simulink model "Full_scale_sim"  (R2024b)
settings: Solver=VariableStepAuto  StartTime=0.0  StopTime=60  RelTol=1e-3
values from neighbouring files (symbols this model uses):
  A_adrcl = [zeros(N, 1)  eye(N, N) ... (first row only)    [Control_Full_Scale_init_example_single_blade_installation.m]
  A_o = [A_m e_m*c_T_d_m ... (first row only)    [Control_Full_Scale_init_example_single_blade_installation.m]
  A_o_lqr = [A_m_lqr e_m*c_T_d_m_lqr ... (first row only)    [Control_Full_Scale_init_example_single_blade_installation.m]
  A_o_nmlqr = [A_m_nmlqr e_m*c_T_d_m_nmlqr ... (first row only)    [Control_Full_Scale_init_example_single_blade_installation.m]
  A_o_plqr = A_m_lqr    [Control_Full_Scale_init_example_single_blade_installation.m]
  b0 = 9.345442381739944e-04    (= 0.000934544238174)    [Control_Full_Scale_init_example_single_blade_installation.m]
  b_adrcl = [zeros(N-1, 1) ... (first row only)    [Control_Full_Scale_init_example_single_blade_installation.m]
  b_o = [b_m ... (first row only)    [Control_Full_Scale_init_example_single_blade_installation.m]
  b_o_lqr = [b_m_lqr ... (first row only)    [Control_Full_Scale_init_example_single_blade_installation.m]
  b_o_nmlqr = [b_m_nmlqr ... (first row only)    [Control_Full_Scale_init_example_single_blade_installation.m]
  b_o_plqr = b_m_lqr    [Control_Full_Scale_init_example_single_blade_installation.m]
  c_o_T = [c_T_m 0]    [Control_Full_Scale_init_example_single_blade_installation.m]
  c_o_T_lqr = [c_T_m_lqr 0]    [Control_Full_Scale_init_example_single_blade_installation.m]
  c_o_T_nmlqr = [c_T_m_nmlqr 0]    [Control_Full_Scale_init_example_single_blade_installation.m]
  c_o_T_plqr = c_T_m_lqr    [Control_Full_Scale_init_example_single_blade_installation.m]
  c_t = [1, zeros(1, N)]    [Control_Full_Scale_init_example_single_blade_installation.m]
  damping_en = 1    [Control_Full_Scale_init_example_single_blade_installation.m]
  eta_init_n = [p_init_n;Theta_init_n]    [Control_Full_Scale_init_example_single_blade_installation.m]
  k = ones(N,1)    [Control_Full_Scale_init_example_single_blade_installation.m]
  k_c_T = acker(A_m,b_m, [-omega_cl,-omega_cl])    [Control_Full_Scale_init_example_single_blade_installation.m]
  k_c_T_lqr = lqr(A_m_lqr,b_m_lqr,Q,R)    [Control_Full_Scale_init_example_single_blade_installation.m]
  k_c_T_nmlqr = lqr(A_m_nmlqr,b_m_nmlqr,Q,R)    [Control_Full_Scale_init_example_single_blade_installation.m]
  k_d_T = (e_m*c_T_d_m) \ b_m    [Control_Full_Scale_init_example_single_blade_installation.m]
  k_d_T_lqr = (e_m*c_T_d_m_lqr) \ b_m_lqr    [Control_Full_Scale_init_example_single_blade_installation.m]
  k_d_T_nmlqr = (e_m*c_T_d_m_nmlqr) \ b_m_nmlqr    [Control_Full_Scale_init_example_single_blade_installation.m]
  k_o = acker(A_o',c_o_T',[-omega_O,-omega_O,-omega_O])'    [Control_Full_Scale_init_example_single_blade_installation.m]
  k_o_lqr = acker(A_o_lqr',c_o_T_lqr',[-omega_O,-omega_O,-omega_O])'    [Control_Full_Scale_init_example_single_blade_installation.m]
  k_o_nmlqr = acker(A_o_nmlqr',c_o_T_nmlqr',[-omega_O,-omega_O,-omega_O])'    [Control_Full_Scale_init_example_single_blade_installation.m]
  k_o_plqr = acker(A_o_plqr',c_o_T_plqr',[-omega_O,-omega_O])'    [Control_Full_Scale_init_example_single_blade_installation.m]
  k_plqr = lqr(A_m_lqr, b_m_lqr, Q, R)    [Control_Full_Scale_init_example_single_blade_installation.m]
  k_s = -inv(c_T_m*inv(A_m-b_m*k_c_T)*b_m)    [Control_Full_Scale_init_example_single_blade_installation.m]
  k_s_lqr = -inv(c_T_m_lqr*inv(A_m_lqr-b_m_lqr*k_c_T_lqr)*b_m_lqr)    [Control_Full_Scale_init_example_single_blade_installation.m]
  k_s_nmlqr = -inv(c_T_m_nmlqr*inv(A_m_nmlqr-b_m_nmlqr*k_c_T_nmlqr)*b_m_nmlqr)    [Control_Full_Scale_init_example_single_blade_installation.m]
  k_s_plqr = -inv(c_T_m*inv(A_m-b_m*k_plqr)*b_m)    [Control_Full_Scale_init_example_single_blade_installation.m]
  k_w1 = gamma * EA/lw1_init    (= 68722339.2973)    [Control_Full_Scale_init_example_single_blade_installation.m]
  k_w2 = 1e8    (= 100000000)    [Control_Full_Scale_init_example_single_blade_installation.m]
  l = ones(N+1, 1)    [Control_Full_Scale_init_example_single_blade_installation.m]
  LADRC_max_effort = 900    [Control_Full_Scale_init_example_single_blade_installation.m]
  lw2 = norm(p_h_init- posSling_n(:,1))-elong_lw2    [Control_Full_Scale_init_example_single_blade_installation.m]
  meanWindSpeed = 12    [Control_Full_Scale_init_example_single_blade_installation.m]
  N = 2    [Control_Full_Scale_init_example_single_blade_installation.m]
  nu_init_b = zeros(6,1)    [Control_Full_Scale_init_example_single_blade_installation.m]
  pitch_damping = 100e+3    (= 100000)    [Control_Full_Scale_init_example_single_blade_installation.m]
  posCraneTip = [0;0;-110]    [Control_Full_Scale_init_example_single_blade_installation.m]
  posSling_b = [bladePar.posCOG + [slings_p1_new(1); -4.5; slings_p1_new(2)],                 bladePar.posCOG + [slings_p1_new(1); 4.5; slings_p1_new(2)],                bladePar.posCOG + [slings_p2_new(1); -4.5; slings_p2_new(2)],                bladePar.posCOG + [slings_p2_new(1); 4.5; slings_p2_new(2)]]    [Control_Full_Scale_init_example_single_blade_installation.m]
  posTuggerline_b = [bladePar.posCOG+[0;-4.5;0],bladePar.posCOG+[0;-35;0]]    [Control_Full_Scale_init_example_single_blade_installation.m]
undefined symbols (not defined in the file or in its folder): bladePar, k_T_d, sigbuilder_block
libraries: MarIn_blade x24, simulink_extras x3, vrlib x3, slpidlib x2, dspstat3 x1
(part 1 of 2)
settings Model: Creator=Basti  LastModifiedBy=Henrik
settings DebuggingCC: UnconnectedInputMsg=warning  UnconnectedOutputMsg=warning  UnconnectedLineMsg=warning
settings ModelReferenceCC: EnableRefExpFcnMdlSchedulingChecks=on
settings RTWCC: GPUComputeCapability=3.5  DLArmComputeVersion=19.05

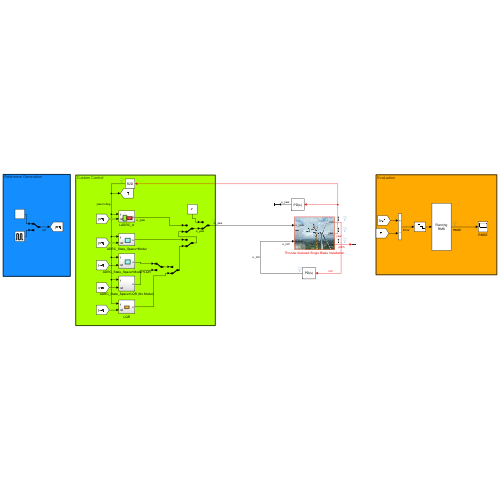
[thumbnail: Simulink's stored preview of the top-level diagram]
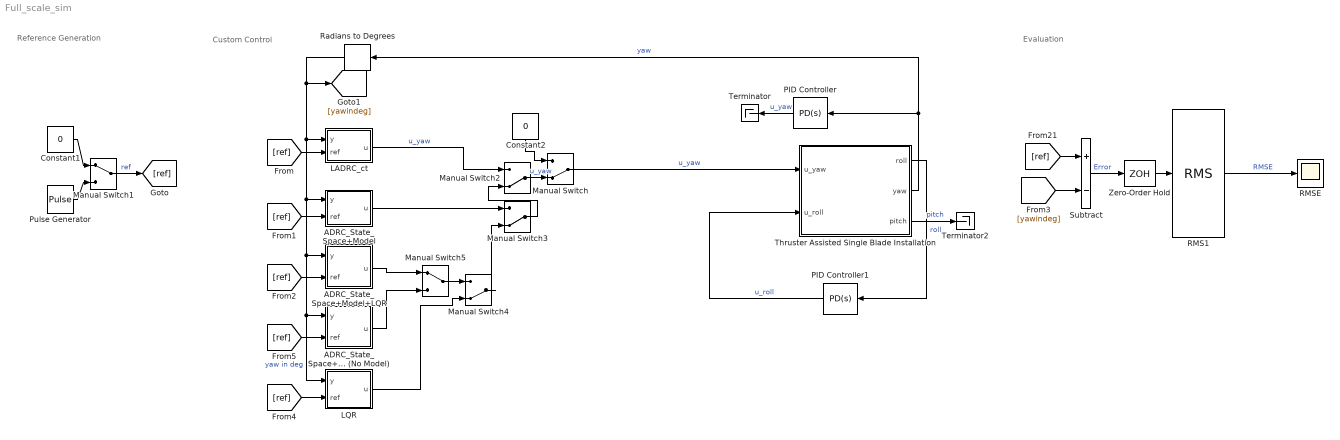
== system Full_scale_sim ==
  note: Evaluation
  note: Reference Generation
  note: Custom Control
  ADRC_State_Space+LQR (No Model) : Subsystem
  ADRC_State_Space+Model : Subsystem
  ADRC_State_Space+Model+LQR : Subsystem
  Constant1 : Constant  Value=0
  Constant2 : Constant  Value=0
  LADRC_ct : Subsystem
  LQR : Subsystem
  Manual Switch{,2..4} (4 alike) : ManualSwitch  CurrentSetting=0
  Manual Switch1 : ManualSwitch
  Manual Switch5 : ManualSwitch
  PID Controller : slpidlib/PID Controller  Controller=PD  Form=Parallel  TimeDomain=Continuous-time  UseExternalTs=off  SampleTime=-1  IntegratorMethod=Forward Euler  FilterMethod=Forward Euler  ControllerParametersSource=internal  P=5000  I=0  UseKiTs=off  D=35414.6651049002  UseExternalDerivativeSource=off  N=35.5205953021552  UseFilter=on  TunerSelectOption=Transfer Function Based (PID Tuner App)  InitialConditionSource=internal  InitialConditionForIntegrator=0  InitialConditionForFilter=0  DifferentiatorICPrevScaledInput=0  ExternalReset=none  TrackingMode=off  Kt=1  LimitOutput=off  SatLimitsSource=internal  UpperSaturationLimit=inf  LowerSaturationLimit=-inf  LinearizeAsGain=on  AntiWindupMode=none  Kb=1  LimitIntegrator=off  UpperIntegratorSaturationLimit=inf  LowerIntegratorSaturationLimit=-inf  POutMin=[]  POutMax=[]  IOutMin=[]  IOutMax=[]  DOutMin=[]  DOutMax=[]  NOutMin=[]  NOutMax=[]  SumOutMin=[]  SumOutMax=[]  SaturationOutMin=[]  SaturationOutMax=[]  PParamMin=[]  PParamMax=[]  IParamMin=[]  IParamMax=[]  DParamMin=[]  DParamMax=[]  NParamMin=[]  NParamMax=[]  KbParamMin=[]  KbParamMax=[]  KtParamMin=[]  KtParamMax=[]  KbOutMin=[]  KbOutMax=[]  KtOutMin=[]  KtOutMax=[]  IntegratorOutMin=[]  IntegratorOutMax=[]  FilterOutMin=[]  FilterOutMax=[]  SumI1OutMin=[]  SumI1OutMax=[]  SumI2OutMin=[]  SumI2OutMax=[]  SumI3OutMin=[]  SumI3OutMax=[]  SumI4OutMin=[]  SumI4OutMax=[]  SumDOutMin=[]  SumDOutMax=[]  DifferentiatorOutMin=[]  DifferentiatorOutMax=[]  FilterDiffOutCoefMin=[]  FilterDiffOutCoefMax=[]  ReciprocalOutMin=[]  ReciprocalOutMax=[]  SumDenOutMin=[]  SumDenOutMax=[]  SumNumOutMin=[]  SumNumOutMax=[]  DivideOutMin=[]  DivideOutMax=[]  UdiffTsProdOutMin=[]  UdiffTsProdOutMax=[]  NTsProdOutMin=[]  NTsProdOutMax=[]  UintegralTsProdOutMin=[]  UintegralTsProdOutMax=[]  UngainTsProdOutMin=[]  UngainTsProdOutMax=[]  ClampingZeroOutDataTypeStr=Inherit: Inherit via back propagation  ClampingZeroOutMin=[]  ClampingZeroOutMax=[]  FilterDenConstantOutDataTypeStr=Inherit: Inherit via back propagation  FilterDenConstantOutMin=[]  FilterDenConstantOutMax=[]  PCopyOutDataTypeStr=Inherit: Inherit via back propagation  PCopyOutMin=[]  PCopyOutMax=[]  NCopyOutDataTypeStr=Inherit: Inherit via back propagation  NCopyOutMin=[]  NCopyOutMax=[]  IntegratorContinuousStateAttributes=''  IntegratorStateMustResolveToSignalObject=off  IntegratorRTWStateStorageClass=Auto  FilterContinuousStateAttributes=''  FilterStateMustResolveToSignalObject=off  FilterRTWStateStorageClass=Auto  ParallelPVariant=InternalParameters  IdealPVariant=Disabled  IVariant=Disabled  DVariant=InternalParameters  IntegratorVariant=Disabled  SatVariant=Disabled  AWVariant=Disabled  PCopyVariant=Disabled  TRVariant=Disabled  FdbkBlocksVariant=Forward  IdealPFdbkVariant=Disabled  SatFdbkVariant=Disabled  DerivativeFilterVariant=ContFilter  NVariant=InternalParameters  NCopyVariant=Disabled  FilterICVariant=InternalICsFilter  IntegratorICVariant=Disabled  ExternalResetVariant=Disabled  TRSumVariant=Passthrough  SumFdbkVariant=Disabled  SumVariant=Sum_PD  TsampFilterVariant=InternalTs  TsampNgainVariant=Passthrough  TsampIntegralVariant=Disabled_SignalSpec  ExternalSaturationOutDataTypeStr=Inherit: Same as second input  DerivativeSourceVariant=ErrorSignal  PreIntVariant=InternalPreInt
  PID Controller1 : slpidlib/PID Controller  Controller=PD  Form=Parallel  TimeDomain=Continuous-time  UseExternalTs=off  SampleTime=-1  IntegratorMethod=Forward Euler  FilterMethod=Forward Euler  ControllerParametersSource=internal  P=200  I=0  UseKiTs=off  D=300000  UseExternalDerivativeSource=off  N=100  UseFilter=on  TunerSelectOption=Transfer Function Based (PID Tuner App)  InitialConditionSource=internal  InitialConditionForIntegrator=0  InitialConditionForFilter=0  DifferentiatorICPrevScaledInput=0  ExternalReset=none  TrackingMode=off  Kt=1  LimitOutput=off  SatLimitsSource=internal  UpperSaturationLimit=inf  LowerSaturationLimit=-inf  LinearizeAsGain=on  AntiWindupMode=none  Kb=1  LimitIntegrator=off  UpperIntegratorSaturationLimit=inf  LowerIntegratorSaturationLimit=-inf  POutMin=[]  POutMax=[]  IOutMin=[]  IOutMax=[]  DOutMin=[]  DOutMax=[]  NOutMin=[]  NOutMax=[]  SumOutMin=[]  SumOutMax=[]  SaturationOutMin=[]  SaturationOutMax=[]  PParamMin=[]  PParamMax=[]  IParamMin=[]  IParamMax=[]  DParamMin=[]  DParamMax=[]  NParamMin=[]  NParamMax=[]  KbParamMin=[]  KbParamMax=[]  KtParamMin=[]  KtParamMax=[]  KbOutMin=[]  KbOutMax=[]  KtOutMin=[]  KtOutMax=[]  IntegratorOutMin=[]  IntegratorOutMax=[]  FilterOutMin=[]  FilterOutMax=[]  SumI1OutMin=[]  SumI1OutMax=[]  SumI2OutMin=[]  SumI2OutMax=[]  SumI3OutMin=[]  SumI3OutMax=[]  SumI4OutMin=[]  SumI4OutMax=[]  SumDOutMin=[]  SumDOutMax=[]  DifferentiatorOutMin=[]  DifferentiatorOutMax=[]  FilterDiffOutCoefMin=[]  FilterDiffOutCoefMax=[]  ReciprocalOutMin=[]  ReciprocalOutMax=[]  SumDenOutMin=[]  SumDenOutMax=[]  SumNumOutMin=[]  SumNumOutMax=[]  DivideOutMin=[]  DivideOutMax=[]  UdiffTsProdOutMin=[]  UdiffTsProdOutMax=[]  NTsProdOutMin=[]  NTsProdOutMax=[]  UintegralTsProdOutMin=[]  UintegralTsProdOutMax=[]  UngainTsProdOutMin=[]  UngainTsProdOutMax=[]  ClampingZeroOutDataTypeStr=Inherit: Inherit via back propagation  ClampingZeroOutMin=[]  ClampingZeroOutMax=[]  FilterDenConstantOutDataTypeStr=Inherit: Inherit via back propagation  FilterDenConstantOutMin=[]  FilterDenConstantOutMax=[]  PCopyOutDataTypeStr=Inherit: Inherit via back propagation  PCopyOutMin=[]  PCopyOutMax=[]  NCopyOutDataTypeStr=Inherit: Inherit via back propagation  NCopyOutMin=[]  NCopyOutMax=[]  IntegratorContinuousStateAttributes=''  IntegratorStateMustResolveToSignalObject=off  IntegratorRTWStateStorageClass=Auto  FilterContinuousStateAttributes=''  FilterStateMustResolveToSignalObject=off  FilterRTWStateStorageClass=Auto  ParallelPVariant=InternalParameters  IdealPVariant=Disabled  IVariant=Disabled  DVariant=InternalParameters  IntegratorVariant=Disabled  SatVariant=Disabled  AWVariant=Disabled  PCopyVariant=Disabled  TRVariant=Disabled  FdbkBlocksVariant=Forward  IdealPFdbkVariant=Disabled  SatFdbkVariant=Disabled  DerivativeFilterVariant=ContFilter  NVariant=InternalParameters  NCopyVariant=Disabled  FilterICVariant=InternalICsFilter  IntegratorICVariant=Disabled  ExternalResetVariant=Disabled  TRSumVariant=Passthrough  SumFdbkVariant=Disabled  SumVariant=Sum_PD  TsampFilterVariant=InternalTs  TsampNgainVariant=Passthrough  TsampIntegralVariant=Disabled_SignalSpec  ExternalSaturationOutDataTypeStr=Inherit: Same as second input  DerivativeSourceVariant=ErrorSignal  PreIntVariant=InternalPreInt
  Pulse Generator : DiscretePulseGenerator  PulseType=Time based  Amplitude=90  Period=40  PulseWidth=50
  RMS1 : dspstat3/RMS  run=on  directionMode=Entire input  dimension=1  reset_popup=None
  RMSE : Scope
  Radians to Degrees : simulink_extras/Transformations/Radians to Degrees
  Subtract : Sum  Inputs=+-
  Terminator : Terminator
  Terminator2 : Terminator
  Thruster Assisted Single Blade Installation : Subsystem  AncestorBlock=MarIn_blade/[Example] Single blade installation  mask([Example] Single blade installation){}
      mask help:
      | This is an example to use the MarIn toolbox to model single blade installation.
      |
      | Author: Zhengru Ren
      | Date:  19/09/2017
      mask Display: image('apsicon.png');
  Zero-Order Hold : ZeroOrderHold  SampleTime=0.5
  wires:
  Thruster Assisted Single Blade Installation/3(pitch) -> Terminator2/1  "pitch"
  Thruster Assisted Single Blade Installation/2(yaw) -> Radians to Degrees/1, PID Controller/1  "yaw"
  PID Controller1/1 -> Thruster Assisted Single Blade Installation/2(u_roll)  "u_roll"
  Thruster Assisted Single Blade Installation/1(roll) -> PID Controller1/1  "roll"
  Manual Switch/1 -> Thruster Assisted Single Blade Installation/1(u_yaw)  "u_yaw"
  PID Controller/1 -> Terminator/1  "u_yaw"
  Radians to Degrees/1 -> LQR/1(y), ADRC_State_Space+LQR (No Model)/1(y), ADRC_State_Space+Model+LQR/1(y), ADRC_State_Space+Model/1(y), LADRC_ct/1(y), [yawindeg]  "yaw in deg"
  LADRC_ct/1(u) -> Manual Switch2/1  "u_yaw"
  ADRC_State_Space+Model/1(u) -> Manual Switch3/1
  Constant1/1 -> Manual Switch1/1
  Pulse Generator/1 -> Manual Switch1/2
  Manual Switch2/1 -> Manual Switch/2  "u_yaw"
  Constant2/1 -> Manual Switch/1
  Subtract/1 -> Zero-Order Hold/1  "Error"
  [ref] -> Subtract/1
  RMS1/1 -> RMSE/1  "RMSE"
  Manual Switch1/1 -> [ref]  "ref"
  [ref] -> LADRC_ct/2(ref)
  [ref] -> ADRC_State_Space+Model/2(ref)
  [ref] -> ADRC_State_Space+Model+LQR/2(ref)
  ADRC_State_Space+Model+LQR/1(u) -> Manual Switch5/1
  Manual Switch3/1 -> Manual Switch2/2
  Zero-Order Hold/1 -> RMS1/1
  [yawindeg] -> Subtract/2
  [ref] -> LQR/2(ref)
  LQR/1(u) -> Manual Switch4/2
  Manual Switch4/1 -> Manual Switch3/2
  [ref] -> ADRC_State_Space+LQR (No Model)/2(ref)
  ADRC_State_Space+LQR (No Model)/1(u) -> Manual Switch5/2
  Manual Switch5/1 -> Manual Switch4/1

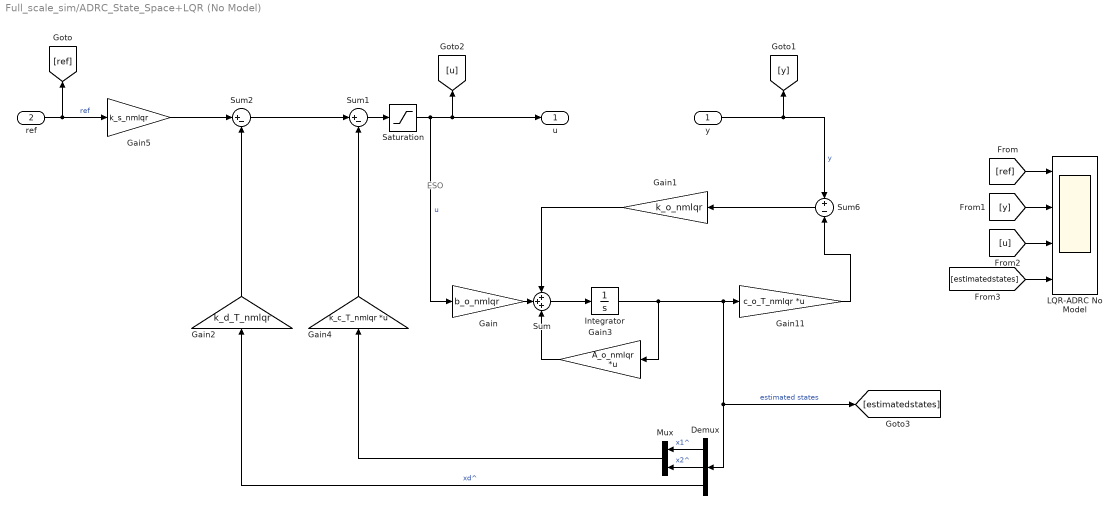
== system Full_scale_sim/ADRC_State_Space+LQR (No Model) ==
  note: ESO
  y : Inport
  ref : Inport  Port=2
  Demux : Demux  Outputs=N+1
  Gain : Gain  Gain=b_o_nmlqr
  Gain1 : Gain  Gain=k_o_nmlqr
  Gain11 : Gain  Gain=c_o_T_nmlqr  Multiplication=Matrix(K*u)
  Gain2 : Gain  Gain=k_d_T_nmlqr
  Gain3 : Gain  Gain=A_o_nmlqr  Multiplication=Matrix(K*u)
  Gain4 : Gain  Gain=k_c_T_nmlqr  Multiplication=Matrix(K*u)
  Gain5 : Gain  Gain=k_s_nmlqr
  Integrator : Integrator
  LQR-ADRC No Model : Scope  NumInputPorts=4
  Mux : Mux  Inputs=2
  Saturation : Saturate  UpperLimit=LADRC_max_effort  LowerLimit=-LADRC_max_effort
  Sum : Sum  Inputs=+++
  Sum1 : Sum  Inputs=|+-
  Sum2 : Sum  Inputs=|+-
  Sum6 : Sum  Inputs=+|-
  u : Outport
  wires:
  Gain5/1 -> Sum2/1
  Sum2/1 -> Sum1/1
  Gain2/1 -> Sum2/2
  Gain4/1 -> Sum1/2
  Mux/1 -> Gain4/1
  Sum1/1 -> Saturation/1
  Demux/3 -> Gain2/1  "xd^"
  Demux/2 -> Mux/2  "x2^"
  Demux/1 -> Mux/1  "x1^"
  Gain3/1 -> Sum/3
  Sum/1 -> Integrator/1
  Gain1/1 -> Sum/1
  Gain/1 -> Sum/2
  Sum6/1 -> Gain1/1
  [estimatedstates] -> LQR-ADRC No Model/4
  [u] -> LQR-ADRC No Model/3
  [y] -> LQR-ADRC No Model/2
  [ref] -> LQR-ADRC No Model/1
  y/1 -> [y], Sum6/1  "y"
  ref/1 -> [ref], Gain5/1  "ref"
  Gain11/1 -> Sum6/2
  Integrator/1 -> Gain11/1, Demux/1, [estimatedstates], Gain3/1  "estimated states"
  Saturation/1 -> u/1, [u], Gain/1  "u"

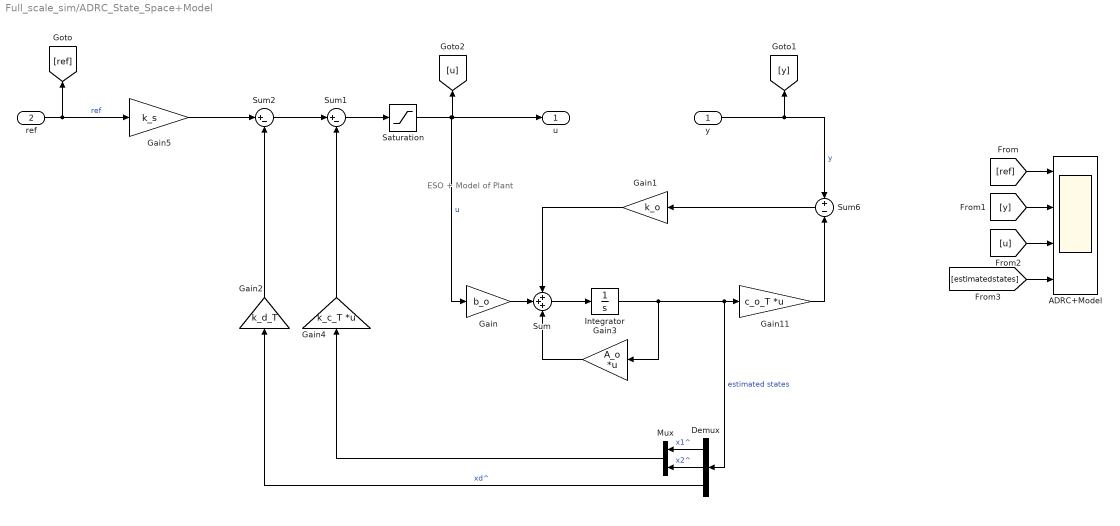
== system Full_scale_sim/ADRC_State_Space+Model ==
  note: ESO + Model of Plant
  y : Inport
  ref : Inport  Port=2
  ADRC+Model : Scope  NumInputPorts=4
  Demux : Demux  Outputs=N+1
  Gain : Gain  Gain=b_o
  Gain1 : Gain  Gain=k_o
  Gain11 : Gain  Gain=c_o_T  Multiplication=Matrix(K*u)
  Gain2 : Gain  Gain=k_d_T
  Gain3 : Gain  Gain=A_o  Multiplication=Matrix(K*u)
  Gain4 : Gain  Gain=k_c_T  Multiplication=Matrix(K*u)
  Gain5 : Gain  Gain=k_s
  Integrator : Integrator
  Mux : Mux  Inputs=2
  Saturation : Saturate  UpperLimit=LADRC_max_effort  LowerLimit=-LADRC_max_effort
  Sum : Sum  Inputs=+++
  Sum1 : Sum  Inputs=|+-
  Sum2 : Sum  Inputs=|+-
  Sum6 : Sum  Inputs=+|-
  u : Outport
  wires:
  Saturation/1 -> [u], u/1, Gain/1  "u"
  Integrator/1 -> Gain3/1, Demux/1, Gain11/1  "estimated states"
  Gain11/1 -> Sum6/2
  ref/1 -> Gain5/1, [ref]  "ref"
  y/1 -> Sum6/1, [y]  "y"
  [ref] -> ADRC+Model/1
  [y] -> ADRC+Model/2
  [u] -> ADRC+Model/3
  [estimatedstates] -> ADRC+Model/4
  Sum6/1 -> Gain1/1
  Gain/1 -> Sum/2
  Gain1/1 -> Sum/1
  Sum/1 -> Integrator/1
  Gain3/1 -> Sum/3
  Demux/1 -> Mux/1  "x1^"
  Demux/2 -> Mux/2  "x2^"
  Demux/3 -> Gain2/1  "xd^"
  Sum1/1 -> Saturation/1
  Mux/1 -> Gain4/1
  Gain4/1 -> Sum1/2
  Gain2/1 -> Sum2/2
  Sum2/1 -> Sum1/1
  Gain5/1 -> Sum2/1

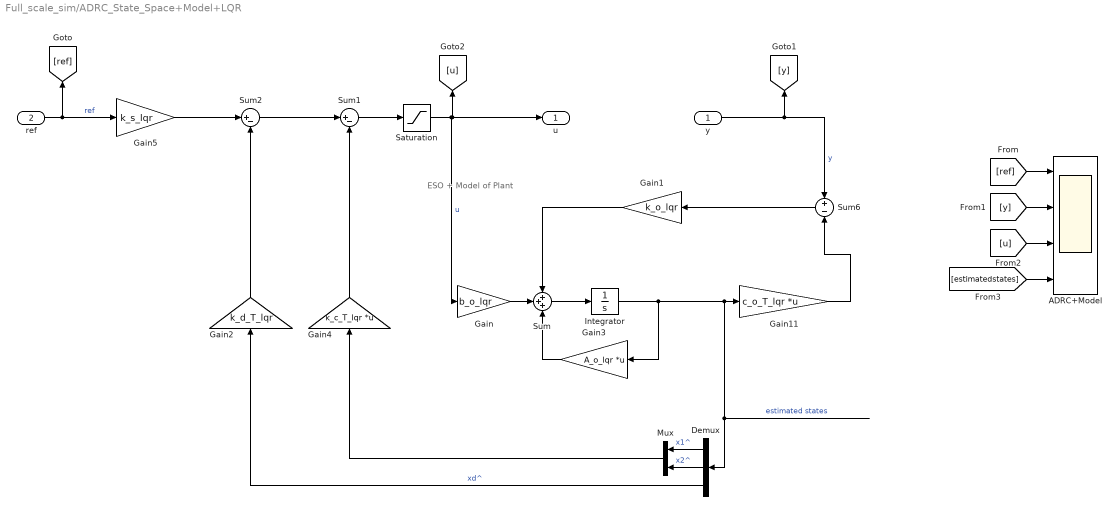
== system Full_scale_sim/ADRC_State_Space+Model+LQR ==
  note: ESO + Model of Plant
  y : Inport
  ref : Inport  Port=2
  ADRC+Model : Scope  NumInputPorts=4
  Demux : Demux  Outputs=N+1
  Gain : Gain  Gain=b_o_lqr
  Gain1 : Gain  Gain=k_o_lqr
  Gain11 : Gain  Gain=c_o_T_lqr  Multiplication=Matrix(K*u)
  Gain2 : Gain  Gain=k_d_T_lqr
  Gain3 : Gain  Gain=A_o_lqr  Multiplication=Matrix(K*u)
  Gain4 : Gain  Gain=k_c_T_lqr  Multiplication=Matrix(K*u)
  Gain5 : Gain  Gain=k_s_lqr
  Integrator : Integrator
  Mux : Mux  Inputs=2
  Saturation : Saturate  UpperLimit=LADRC_max_effort  LowerLimit=-LADRC_max_effort
  Sum : Sum  Inputs=+++
  Sum1 : Sum  Inputs=|+-
  Sum2 : Sum  Inputs=|+-
  Sum6 : Sum  Inputs=+|-
  u : Outport
  wires:
  Saturation/1 -> [u], u/1, Gain/1  "u"
  Integrator/1 -> Gain3/1, Demux/1, Gain11/1  "estimated states"
  Gain11/1 -> Sum6/2
  ref/1 -> Gain5/1, [ref]  "ref"
  y/1 -> Sum6/1, [y]  "y"
  [ref] -> ADRC+Model/1
  [y] -> ADRC+Model/2
  [u] -> ADRC+Model/3
  [estimatedstates] -> ADRC+Model/4
  Sum6/1 -> Gain1/1
  Gain/1 -> Sum/2
  Gain1/1 -> Sum/1
  Sum/1 -> Integrator/1
  Gain3/1 -> Sum/3
  Demux/1 -> Mux/1  "x1^"
  Demux/2 -> Mux/2  "x2^"
  Demux/3 -> Gain2/1  "xd^"
  Sum1/1 -> Saturation/1
  Mux/1 -> Gain4/1
  Gain4/1 -> Sum1/2
  Gain2/1 -> Sum2/2
  Sum2/1 -> Sum1/1
  Gain5/1 -> Sum2/1

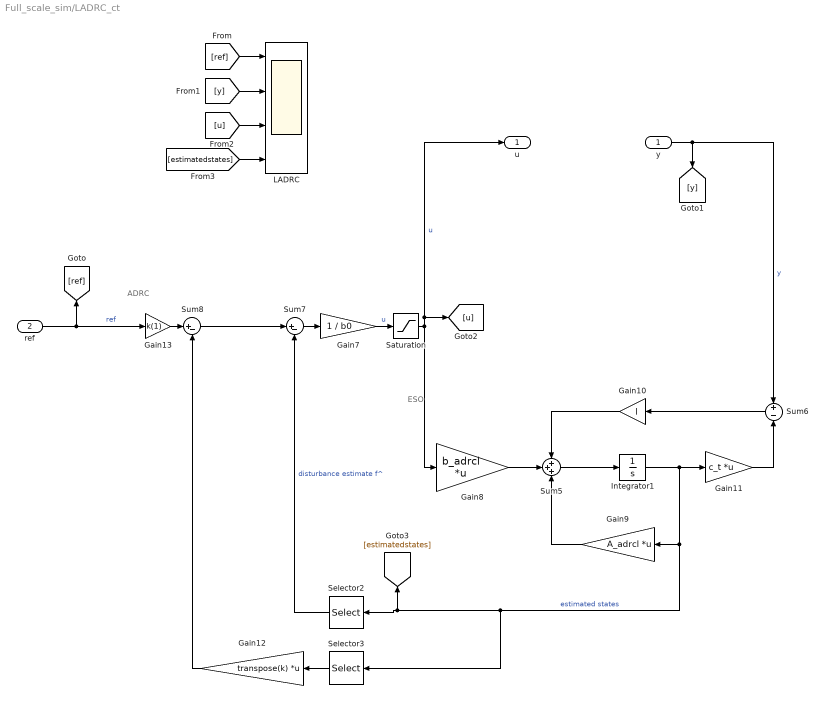
== system Full_scale_sim/LADRC_ct ==
  note: ESO
  note: ADRC
  y : Inport
  ref : Inport  Port=2
  Gain10 : Gain  Gain=l
  Gain11 : Gain  Gain=c_t  Multiplication=Matrix(K*u)
  Gain12 : Gain  Gain=transpose(k)  Multiplication=Matrix(K*u)
  Gain13 : Gain  Gain=k(1)
  Gain7 : Gain  Gain=1 / b0
  Gain8 : Gain  Gain=b_adrcl  Multiplication=Matrix(K*u)
  Gain9 : Gain  Gain=A_adrcl  Multiplication=Matrix(K*u)
  Integrator1 : Integrator
  LADRC : Scope  NumInputPorts=4
  Saturation : Saturate  UpperLimit=LADRC_max_effort  LowerLimit=-LADRC_max_effort
  Selector2 : Selector  InputPortWidth=N+1  IndexOptions=Index vector (dialog)  Indices=[N+1]  OutputSizes=1
  Selector3 : Selector  InputPortWidth=N+1  IndexOptions=Index vector (dialog)  Indices=[1:N]  OutputSizes=1
  Sum5 : Sum  Inputs=+++
  Sum6 : Sum  Inputs=+|-
  Sum7 : Sum  Inputs=|+-
  Sum8 : Sum  Inputs=|+-
  u : Outport
  wires:
  Gain8/1 -> Sum5/2
  Saturation/1 -> u/1, [u], Gain8/1  "u"
  Integrator1/1 -> Gain11/1, Selector3/1, [estimatedstates], Selector2/1, Gain9/1  "estimated states"
  Gain11/1 -> Sum6/2
  Sum6/1 -> Gain10/1
  Selector2/1 -> Sum7/2  "disturbance estimate f^"
  Sum7/1 -> Gain7/1
  Gain12/1 -> Sum8/2
  Gain10/1 -> Sum5/1
  Gain9/1 -> Sum5/3
  Gain13/1 -> Sum8/1
  Sum5/1 -> Integrator1/1
  Selector3/1 -> Gain12/1
  Sum8/1 -> Sum7/1
  ref/1 -> [ref], Gain13/1  "ref"
  y/1 -> Sum6/1, [y]  "y"
  [ref] -> LADRC/1
  [y] -> LADRC/2
  [u] -> LADRC/3
  [estimatedstates] -> LADRC/4
  Gain7/1 -> Saturation/1  "u"

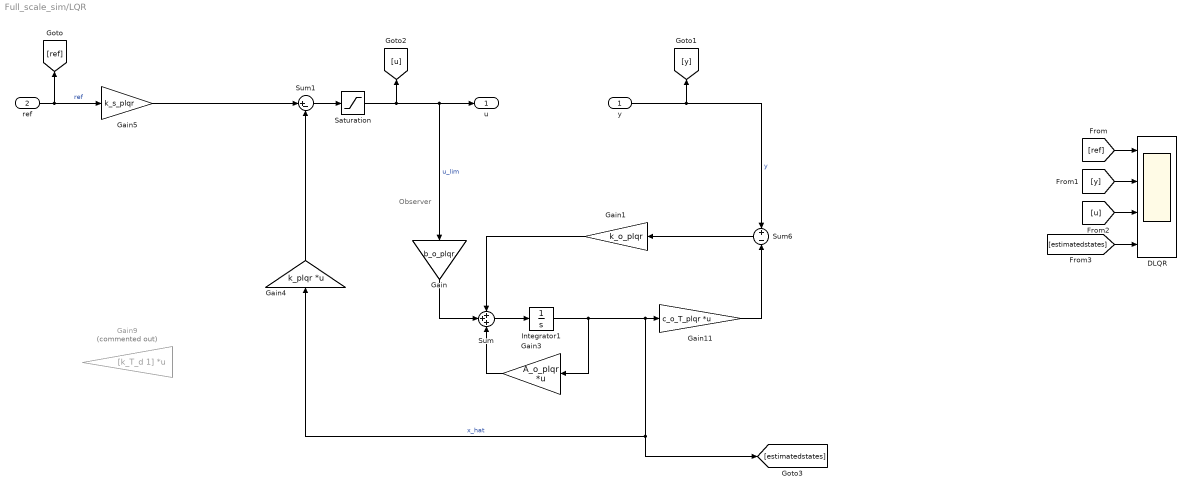
== system Full_scale_sim/LQR ==
  note: Observer
  y : Inport
  ref : Inport  Port=2
  DLQR : Scope  NumInputPorts=4
  Gain : Gain  Gain=b_o_plqr
  Gain1 : Gain  Gain=k_o_plqr
  Gain11 : Gain  Gain=c_o_T_plqr  Multiplication=Matrix(K*u)
  Gain3 : Gain  Gain=A_o_plqr  Multiplication=Matrix(K*u)
  Gain4 : Gain  Gain=k_plqr  Multiplication=Matrix(K*u)
  Gain5 : Gain  Gain=k_s_plqr
  Gain9 : Gain  Commented=on  Gain=[k_T_d 1]  Multiplication=Matrix(K*u)
  Integrator1 : Integrator
  Saturation : Saturate  UpperLimit=LADRC_max_effort  LowerLimit=-LADRC_max_effort
  Sum : Sum  Inputs=+++
  Sum1 : Sum  Inputs=|+-
  Sum6 : Sum  Inputs=+|-
  u : Outport
  wires:
  ref/1 -> Gain5/1, [ref]  "ref"
  [ref] -> DLQR/1
  [y] -> DLQR/2
  [u] -> DLQR/3
  [estimatedstates] -> DLQR/4
  Sum1/1 -> Saturation/1
  Gain4/1 -> Sum1/2
  Gain5/1 -> Sum1/1
  Saturation/1 -> u/1, Gain/1, [u]  "u_lim"
  y/1 -> Sum6/1, [y]  "y"
  Sum6/1 -> Gain1/1
  Sum/1 -> Integrator1/1
  Gain/1 -> Sum/2
  Gain1/1 -> Sum/1
  Gain11/1 -> Sum6/2
  Integrator1/1 -> Gain3/1, [estimatedstates], Gain4/1, Gain11/1  "x_hat"
  Gain3/1 -> Sum/3

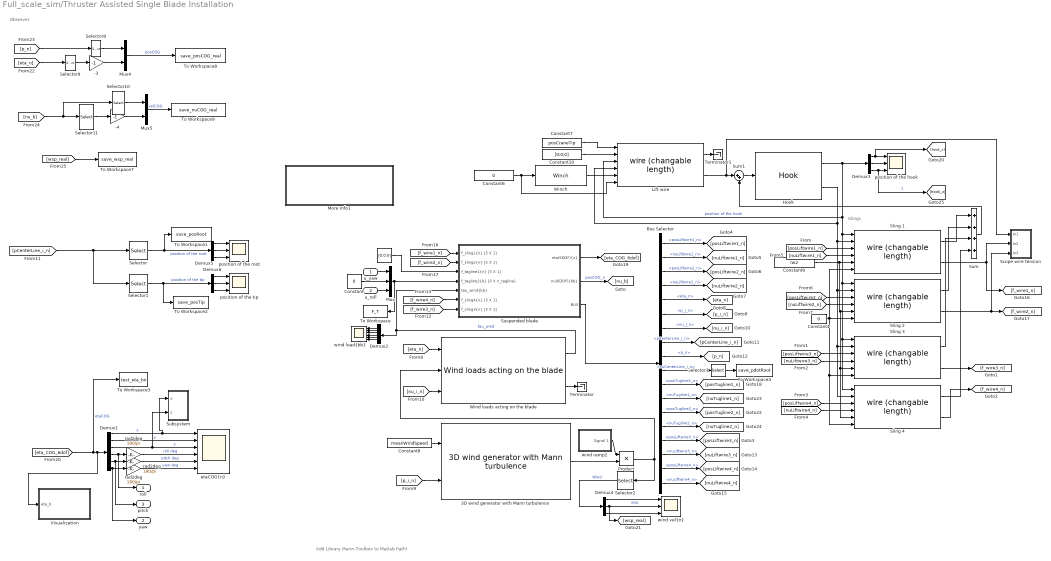
== system Full_scale_sim/Thruster Assisted Single Blade Installation ==
  note: Add Library Marin-Toolbox to Matlab Path!
  note: Slings
  note: Observer
  u_yaw : Inport
  u_roll : Inport  Port=2
  " " : Constant  Value=[0;0;0]
  " rad2deg" : Gain  Gain=180/pi
  -3 : Gain  Gain=-1
  -4 : Gain  Gain=-1
  3D wind generator with Mann turbulence : MarIn_blade/Environment/3D wind generator with Mann turbulence  turbulence_switch=on  posC_tb=[0,0,-90]  angC_tb=[0,0,0]  data_wind_mann=data_wind_mann
      settings: SourceProductName=MarIn (Blade)
  Bus Selector : BusSelector  OutputSignals=posLiftwire1_n,nuLiftwire1_n,posLiftwire2_n,nuLiftwire2_n,eta_n,p_i_n,nu_i_n,pCenterLine_i_n,p_n,nuCenterLine_i_n,posTugline1_n,nuTugline1_n,posTugline2_n,nuTugline2_n,posLiftwire3_n,nuLiftwire3_n,posLiftwire4_n,nuLiftwire4_n
  Constant : Constant  Value=0
  Constant10 : Constant  Value=[0;0;0]
  Constant4 : Constant  Value=0
  Constant6 : Constant  Value=0
  Constant7 : Constant  Value=posCraneTip
  Constant8 : Constant  Value=meanWindSpeed
  Constant9 : Constant  Value=lw2
  Demux1 : Demux  Outputs=6
  Demux2 : Demux  Outputs=6
  Demux{3..6} (4 alike) : Demux  Outputs=3
  Hook : MarIn_blade/Lifting equipments (winch, wire, hook)/Hook  m_h=m_h  p_h_init=p_h_init  p_h_dot_init=p_h_dot_init
      settings: SourceProductName=MarIn (Blade)
  Lift wire : MarIn_blade/Lifting equipments (winch, wire, hook)/wire (changable length)  k=k_w1  c=d_w1
      settings: SourceProductName=MarIn (Blade)
  More Info1 : Subsystem
      settings: OpenFcn=run init_example_single_blade_installation.m
      mask Display: disp('Double-click to initialize the model')
  Mux : Mux  Inputs=3
  Mux4 : Mux  Inputs=2
  Mux5 : Mux  Inputs=2
  Product : Product
  Scope wire tension : Subsystem
  Selector : Selector  NumberOfDimensions=2  InputPortWidth=3  IndexOptions=Index vector (dialog),Index vector (dialog)  Indices=[1 2 3],1  OutputSizes=1,1
  Selector1 : Selector  NumberOfDimensions=2  InputPortWidth=3  IndexOptions=Index vector (dialog),Index vector (dialog)  Indices=[1 2 3],bladePar.n_i  OutputSizes=1,1
  Selector10 : Selector  InputPortWidth=6  IndexOptions=Index vector (dialog)  Indices=[3,2]  OutputSizes=1
  Selector11 : Selector  InputPortWidth=6  IndexOptions=Index vector (dialog)  Indices=4  OutputSizes=1
  Selector2 : Selector  NumberOfDimensions=2  InputPortWidth=3  IndexOptions=Index vector (dialog),Index vector (dialog)  Indices=[1 2 3],20  OutputSizes=1,1
  Selector3 : Selector  NumberOfDimensions=2  InputPortWidth=3  IndexOptions=Index vector (dialog),Index vector (dialog)  Indices=[1 2 3],1  OutputSizes=1,1
  Selector8 : Selector  InputPortWidth=3  IndexOptions=Index vector (dialog)  Indices=[1 2]  OutputSizes=1
  Selector9 : Selector  InputPortWidth=6  IndexOptions=Index vector (dialog)  Indices=4  OutputSizes=1
  Sling {1..4} (4 alike) : MarIn_blade/Lifting equipments (winch, wire, hook)/wire (changable length)  k=k_w2  c=d_w2
      settings: SourceProductName=MarIn (Blade)
  Subsystem : Subsystem
  Sum : Sum  Inputs=++++
  Sum1 : Sum  Inputs=|++
  Suspended blade : Subsystem  AncestorBlock=MarIn_blade/Payload/Suspended blade  mask(Blade){m_yoke=20e3, bladePar=bladePar, eta_init_n=eta_init_n, eta_init_b=nu_init_b, n_tugline=2, posTuggerline_b=posTuggerline_b, n_sling=2, posSling_b=posSling_b}
      mask prompts: m_yoke "Mass of yoke (kg)"; bladePar "Blade parameter structure"; eta_init_n "Initial position and attitude {n}"; eta_init_b "Initial velocity {b}"; n_tugline "Number of tugger lines (n_tugline)"; posTuggerline_b "Position of connection points to the Tuggerlines{b} [n_tugline x 3]"; n_sling "Number of slings (n_sling)"; posSling_b "Position of connection points to the slings {b} [3Xn_sling]"
      mask help:
      | This block is used to simulate a suspended blade lifted by a crane and control by tuglines.
      |
      |
      | Author: Zhengru Ren
      | Date: April 20, 2017
      mask init:
      | invM_total = inv(bladePar.M+diag([m_yoke,m_yoke,m_yoke,0,0,0]));
      mask DialogControl Container6 Prompt: Yoke
      mask DialogControl Container3 Prompt: Blade
      mask DialogControl Container4 Prompt: Tugger lines
      mask DialogControl Container5 Prompt: Lifting wire rope
      mask Display:
      | image(imread('fig/blade.png'))
      | 
      | port_label('input', 1, 'f_sling1{n}')
      | port_label('input', 2, 'f_sling2{n}')
      | port_label('input', 6, 'f_sling4{n}')
      | port_label('input', 7, 'f_sling3{n}')
      | port_label('input', 3, 'f_tagline1{n}')
      | port_label('input', 4, 'f_tagline2{n}')
      | port_label('input', 5, 'tau_wind{b}')
      | 
      | port_label('output', 1, 'etaCOG(6DOF){n}')
      | port_label('output', 2, 'nuCOG(6DOF){b}')
      | port_label('output', 3, 'BUS')
  Terminator : Terminator
  Terminator1 : Terminator
  To Workspace : ToWorkspace  VariableName=F_T  SaveFormat=Timeseries  SampleTime=-1
      settings: Decimation=4
  To Workspace1 : ToWorkspace  VariableName=save_posRoot  SaveFormat=Structure With Time  SampleTime=-1
  To Workspace2 : ToWorkspace  VariableName=save_posTip  SaveFormat=Structure With Time  SampleTime=-1
  To Workspace3 : ToWorkspace  VariableName=test_eta_bn  SaveFormat=Structure With Time  SampleTime=-1
  To Workspace4 : ToWorkspace  VariableName=save_pdotRoot  SaveFormat=Structure With Time  SampleTime=-1
  To Workspace7 : ToWorkspace  VariableName=save_wsp_real  SaveFormat=Structure With Time  SampleTime=-1
  To Workspace8 : ToWorkspace  VariableName=save_posCOG_real  SaveFormat=Structure With Time  SampleTime=-1
  To Workspace9 : ToWorkspace  VariableName=save_nuCOG_real  SaveFormat=Structure With Time  SampleTime=-1
  Visualization : Subsystem
  Winch : MarIn_blade/Lifting equipments (winch, wire, hook)/Winch  l_0=lw1_init
      settings: SourceProductName=MarIn (Blade)
  Wind loads acting on the blade : MarIn_blade/Payload/Wind loads acting on the blade
      link override "Wind loads acting on node i/Lift and drag force 2 {b}": SourceBlock=MarIn_blade/Basic functions/Lift and drag force 2 {b}
      settings: SourceProductName=MarIn (Blade)
  "etaCOG{n}" : Scope  NumInputPorts=6
  position of the hook : Scope  NumInputPorts=3
  position of the root : Scope  NumInputPorts=3
  position of the tip : Scope  NumInputPorts=3
  rad2deg : Gain  Gain=180/pi
  "rad2deg " : Gain  Gain=180/pi
  "wind load{bb}" : Scope  NumInputPorts=6
  wind ramp2 : Subsystem  Tag=STV Subsys  LoadFcn=sigbuilder_block('load');  StartFcn=sigbuilder_block('start');  StopFcn=sigbuilder_block('stop');  ClipboardFcn=sigbuilder_block('clipboard');  mask(Sigbuilder block){tuvar=[0:10]}
      mask help: Simulink:masks:SigbuilderBlock_MD
      mask init:
      | if ~strcmp(get_param(bdroot(gcbh),'SimulationStatus'),'stopped') tuvar = sigbuilder_block('maskInit'); end
      settings: CopyFcn=sigbuilder_block('copy');  DeleteFcn=sigbuilder_block('delete');  ModelCloseFcn=sigbuilder_block('modelClose');  PreSaveFcn=sigbuilder_block('preSave');  PauseFcn=sigbuilder_block('pause');  ContinueFcn=sigbuilder_block('continue');  NameChangeFcn=sigbuilder_block('namechange');  OpenFcn=sigbuilder_block('open',[5.4 5.4 1141.2 580.8 ]);  CloseFcn=sigbuilder_block('close');
      mask Display: plot(0, 0, 100, 100,[2, 2, 32, 32, 2], [68, 8, 8, 68, 68],[32, 2], [38, 38], [32, 19, 2],[53, 60, 44], [32, 17, 17, 2],[16, 16, 31, 31]);txt = getActiveGroup(gcbh);text(2, 100, txt,'verticalAlignment', 'top');
  "wind vel{n}" : Scope  NumInputPorts=3
  roll : Outport
  yaw : Outport  Port=2
  pitch : Outport  Port=3
  wires:
  Wind loads acting on the blade/1 -> Suspended blade/5("tau_wind{bb}"), Demux2/1  "tau_wind"
  rad2deg/1 -> "etaCOG{n}"/5  "pitch deg"
  " rad2deg"/1 -> "etaCOG{n}"/6  "yaw deg"
  "rad2deg "/1 -> "etaCOG{n}"/4  "roll deg"
  Demux1/3 -> Subsystem/2(z), "etaCOG{n}"/3  "z"
  Demux1/1 -> Subsystem/1(x), "etaCOG{n}"/1  "x"
  Demux1/2 -> "etaCOG{n}"/2  "y"
  3D wind generator with Mann turbulence/1 -> Product/2
  [wsp_real] -> To Workspace7/1
  [nu_b] -> Selector10/1, Selector11/1
  [p_n] -> Selector8/1
  [eta_n] -> Selector9/1
  Mux4/1 -> To Workspace8/1  "posCOG"
  Mux5/1 -> To Workspace9/1  "velCOG"
  -4/1 -> Mux5/2
  Selector11/1 -> -4/1
  Selector10/1 -> Mux5/1
  -3/1 -> Mux4/2
  Selector8/1 -> Mux4/1
  Selector9/1 -> -3/1
  Bus Selector/14 -> [nuTugline2_n]  "<nuTugline2_n>"
  Bus Selector/12 -> [nuTugline1_n]  "<nuTugline1_n>"
  Bus Selector/13 -> [posTugline2_n]  "<posTugline2_n>"
  Bus Selector/11 -> [posTugline1_n]  "<posTugline1_n>"
  Selector3/1 -> To Workspace4/1
  Bus Selector/10 -> Selector3/1  "<nuCenterLine_i_n>"
  Suspended blade/1("eta(6DOF){n}") -> [eta_COG_6dof]
  [f_wire2_n] -> Suspended blade/2("f_sling2{n} [3 X 1]")
  [f_wire1_n] -> Suspended blade/1("f_sling1{n} [3 X 1]")
  Bus Selector/9 -> [p_n]  "<p_n>"
  Bus Selector/8 -> [pCenterLine_i_n]  "<pCenterLine_i_n>"
  Bus Selector/7 -> [nu_i_n]  "<nu_i_n>"
  Bus Selector/6 -> [p_i_n]  "<p_i_n>"
  Bus Selector/5 -> [eta_n]  "<eta_n>"
  Bus Selector/4 -> [nuLiftwire2_n]  "<nuLiftwire2_n>"
  Bus Selector/3 -> [posLiftwire2_n]  "<posLiftwire2_n>"
  Bus Selector/2 -> [nuLiftwire1_n]  "<nuLiftwire1_n>"
  Bus Selector/1 -> [posLiftwire1_n]  "<posLiftwire1_n>"
  Demux1/6 -> yaw/1, " rad2deg"/1
  Demux4/2 -> "wind vel{n}"/2, [wsp_real]
  wind ramp2/1(Signal 1) -> Product/1
  Product/1 -> Selector2/1, Wind loads acting on the blade/2
  Constant6/1 -> Winch/1, Lift wire/6
  Constant4/1 -> Sling 4/6, Sling 3/6, Sling 1/6, Sling 2/6
  [pCenterLine_i_n] -> Selector/1, Selector1/1
  Selector1/1 -> Demux6/1, To Workspace2/1  "position of the tip"
  Demux6/2 -> position of the tip/2
  Demux6/3 -> position of the tip/3
  Demux6/1 -> position of the tip/1
  Selector/1 -> To Workspace1/1, Demux5/1  "position of the root"
  Demux5/2 -> position of the root/2
  Demux5/3 -> position of the root/3
  Demux5/1 -> position of the root/1
  Selector2/1 -> Demux4/1  "Wind"
  Demux4/3 -> "wind vel{n}"/3
  Demux4/1 -> "wind vel{n}"/1  "wsp"
  Hook/1 -> Demux3/1, Sling 1/1, Sling 4/1, Sling 3/1, Sling 2/1, Lift wire/3  "position of the hook"
  Demux3/2 -> position of the hook/2
  Demux3/1 -> [hook_x], position of the hook/1
  Sum1/1 -> Hook/1
  Lift wire/1 -> Terminator1/1
  Lift wire/2 -> Scope wire tension/1(In1), Sum1/1
  Sum/1 -> Sum1/2
  Constant10/1 -> Lift wire/2
  Constant7/1 -> Lift wire/1
  Constant9/1 -> Sling 4/5, Sling 3/5, Sling 2/5, Sling 1/5
  [nuLiftwire2_n] -> Sling 2/4
  [posLiftwire2_n] -> Sling 2/3
  Sling 2/2 -> Scope wire tension/3(In3), [f_wire2_n]
  Sling 2/1 -> Sum/2
  [nu_i_n] -> Wind loads acting on the blade/3
  Demux2/6 -> "wind load{bb}"/6
  Demux2/5 -> "wind load{bb}"/5
  Demux2/4 -> "wind load{bb}"/4
  Suspended blade/2("nu(6DOF){bb}") -> [nu_b]  "posCOG_n"
  [nuLiftwire1_n] -> Sling 1/4
  Sling 1/2 -> Scope wire tension/2(In2), [f_wire1_n]
  [eta_n] -> Wind loads acting on the blade/1
  [posLiftwire1_n] -> Sling 1/3
  [p_i_n] -> 3D wind generator with Mann turbulence/2
  Suspended blade/3(BUS) -> Bus Selector/1
  Wind loads acting on the blade/2 -> Terminator/1
  Demux2/3 -> "wind load{bb}"/3
  Demux2/2 -> "wind load{bb}"/2
  Demux2/1 -> "wind load{bb}"/1
  Demux1/4 -> roll/1, "rad2deg "/1
  Demux1/5 -> pitch/1, rad2deg/1
  [eta_COG_6dof] -> Visualization/1(eta_b), Demux1/1, To Workspace3/1  "etaCOG"
  Winch/1 -> Lift wire/5
  Sling 1/1 -> Sum/1
  Hook/2 -> Sling 1/2, Sling 4/2, Sling 3/2, Sling 2/2, Lift wire/4
  Constant8/1 -> 3D wind generator with Mann turbulence/1
  " "/1 -> Suspended blade/3("f_tagline1{n} [3 X 1]")
  u_yaw/1 -> Mux/1
  u_roll/1 -> Mux/3
  Constant/1 -> Mux/2
  Mux/1 -> To Workspace/1, Suspended blade/4("f_tagline2{b} [3 X n_tagline]")
  [nuLiftwire3_n] -> Sling 3/4
  [posLiftwire3_n] -> Sling 3/3
  [nuLiftwire4_n] -> Sling 4/4
  [posLiftwire4_n] -> Sling 4/3
  Sling 3/1 -> Sum/3
  Sling 4/1 -> Sum/4
  Sling 3/2 -> [f_wire3_n]
  Sling 4/2 -> [f_wire4_n]
  [f_wire4_n] -> Suspended blade/6("f_sling4{n} [3 X 1]")
  [f_wire3_n] -> Suspended blade/7("f_sling3{n} [3 X 1]")
  Bus Selector/15 -> [posLiftwire3_n]  "<posLiftwire3_n>"
  Bus Selector/16 -> [nuLiftwire3_n]  "<nuLiftwire3_n>"
  Bus Selector/17 -> [posLiftwire4_n]  "<posLiftwire4_n>"
  Bus Selector/18 -> [nuLiftwire4_n]  "<nuLiftwire4_n>"
  Demux3/3 -> [hook_z], position of the hook/3  "z"

== system Full_scale_sim/Thruster Assisted Single Blade Installation/More Info1 ==

== system Full_scale_sim/Thruster Assisted Single Blade Installation/Scope wire tension ==
  In1 : Inport
  In2 : Inport  Port=2
  In3 : Inport  Port=3
  Tension in the ropes : Scope  NumInputPorts=3
  norm : Fcn  Expr=sqrt(u(1)^2+u(2)^2+u(3)^2)
  norm2 : Fcn  Expr=sqrt(u(1)^2+u(2)^2+u(3)^2)
  norm4 : Fcn  Expr=sqrt(u(1)^2+u(2)^2+u(3)^2)
  wires:
  norm4/1 -> Tension in the ropes/3  "tension lift wire 3"
  norm2/1 -> Tension in the ropes/2  "tension lift wire 2"
  norm/1 -> Tension in the ropes/1  "tension lift wire 1"
  In3/1 -> norm4/1
  In2/1 -> norm2/1
  In1/1 -> norm/1

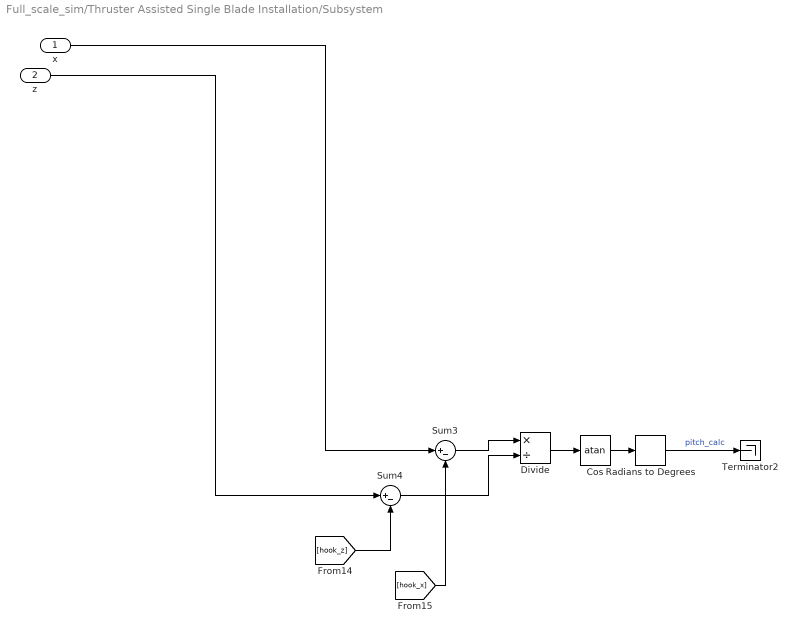
== system Full_scale_sim/Thruster Assisted Single Blade Installation/Subsystem ==
  x : Inport
  z : Inport  Port=2
  Cos : Trigonometry  Operator=atan
  Divide : Product  Inputs=*/
  Radians to Degrees : simulink_extras/Transformations/Radians to Degrees
  Sum3 : Sum  Inputs=|+-
  Sum4 : Sum  Inputs=|+-
  Terminator2 : Terminator
  wires:
  Divide/1 -> Cos/1
  [hook_x] -> Sum3/2
  Cos/1 -> Radians to Degrees/1
  Sum3/1 -> Divide/1
  [hook_z] -> Sum4/2
  Radians to Degrees/1 -> Terminator2/1  "pitch_calc"
  Sum4/1 -> Divide/2
  x/1 -> Sum3/1
  z/1 -> Sum4/1

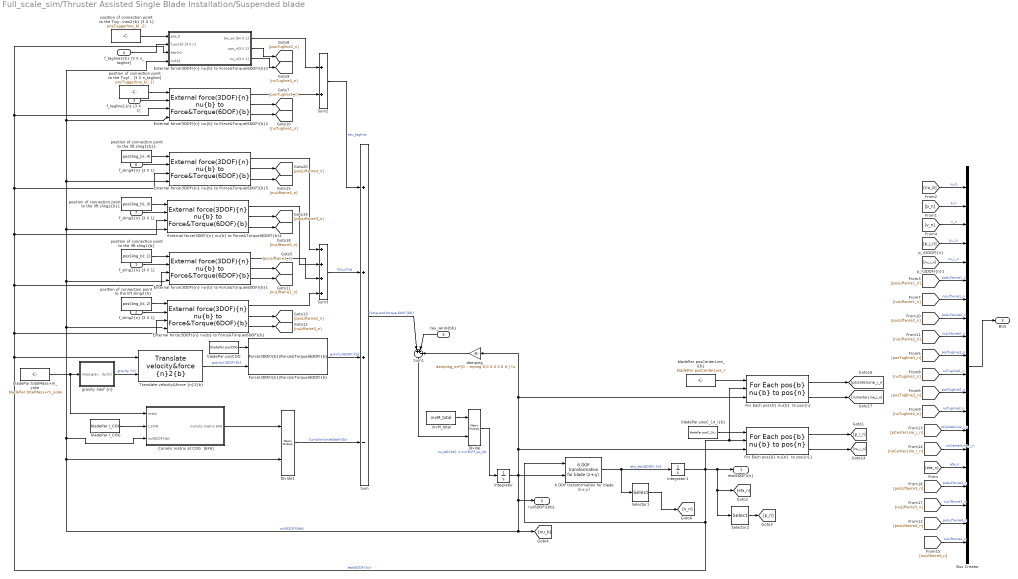
== system Full_scale_sim/Thruster Assisted Single Blade Installation/Suspended blade ==
  "f_sling1{n} [3 X 1]" : Inport
  "f_sling2{n} [3 X 1]" : Inport  Port=2
  "f_tagline1{n} [3 X 1]" : Inport  Port=3
  "f_tagline2{b} [3 X n_tagline]" : Inport  Port=4
  "tau_wind{bb}" : Inport  Port=5
  "f_sling4{n} [3 X 1]" : Inport  Port=6
  "f_sling3{n} [3 X 1]" : Inport  Port=7
  6 DOF transformation for blade (z-x-y) : MarIn_blade/Basic functions/6 DOF transformation for blade (z-x-y)
      settings: SourceProductName=MarIn(Blade)
  Bus Creator : BusCreator  Inputs=20
  Coriolis matrix at COG  [6X6] : Subsystem  AncestorBlock="MarIn_blade/Basic functions/Coriolis matrix at COG  [6X6]"  mask(Mass matrix at COG[6X6]){}
      mask help:
      | This block is used to generate the 6X6 mass matrix at the COG.
      |
      |
      | Author: Zhengru Ren
      | Date: April 20, 2017
  Divide : Product  Inputs=**  Multiplication=Matrix(*)
  Divide1 : Product  Inputs=**  Multiplication=Matrix(*)
  External force(3DOF){n} nu{b} to Force&Torque(6DOF){b}{,1..2,4..5} (5 alike) : MarIn_blade/Basic functions/External force(3DOF){n} nu{b} to Force&Torque(6DOF){b}
      settings: SourceProductName=MarIn(Blade)
  "External force(3DOF){n} nu{b} to Force&Torque(6DOF){b}3" : Subsystem  AncestorBlock=MarIn_blade/Basic functions/External force(3DOF){n} nu{b} to Force&Torque(6DOF){b}  mask(External force(3DOF){n} nu{b} to Force&Torque(6DOF){b}){}
      mask help:
      | Translate position and velocity in {b} to {n}.
      |
      |
      | Author: Zhengru Ren
      | Date: April 22, 2017
  "For Each pos{b} nu{b}  to pos{n}" : MarIn_blade/Basic functions/For Each pos{b} nu{b}  to pos{n}  posCOG_b=bladePar.posCOG  n_i=bladePar.n_i
      settings: SourceProductName=MarIn(Blade)
  "For Each pos{b} nu{b}  to pos{n}1" : MarIn_blade/Basic functions/For Each pos{b} nu{b}  to pos{n}  posCOG_b=bladePar.posCOG  n_i=bladePar.n_i
      settings: SourceProductName=MarIn(Blade)
  "Force(3DOF){b}2Force&Torque(6DOF){b}" : MarIn_blade/Basic functions/Force(3DOF){b}2Force&Torque(6DOF){b}  posCOG_bb=bladePar.posCOG
      settings: SourceProductName=MarIn(Blade)
  Integrator : Integrator  InitialCondition=nu_init_b  ContinuousStateAttributes='nu_b'
  Integrator1 : Integrator  InitialCondition=eta_init_n  ContinuousStateAttributes='eta_n'
  Selector1 : Selector  InputPortWidth=6  IndexOptions=Index vector (dialog)  Indices=[1 2 3]  OutputSizes=1
  Selector2 : Selector  InputPortWidth=6  IndexOptions=Index vector (dialog)  Indices=[1 2 3]  OutputSizes=1
  Sum : Sum  Inputs=+++-
  Sum1 : Sum  Inputs=|++-
  Sum2 : Sum  Inputs=2
  Sum3 : Sum  Inputs=4
  "Translate velocity&force {n}2{b}" : MarIn_blade/Basic functions/Translate velocity&force {n}2{b}
      settings: SourceProductName=MarIn(Blade)
  bladePar.I_COG : Constant  Value=bladePar.I_COG
  bladePar.posCOG : Constant  Value=bladePar.posCOG
  "bladePar.posC_14_i{b}" : Constant  Value=bladePar.posC_14_i
  "bladePar.posCenterLine_i{b}" : Constant  Value=bladePar.posCenterLine_i'
  bladePar.totalMass+m_yoke : Constant  Value=bladePar.totalMass+m_yoke
  damping : Gain  Gain=damping_en*[0 0 0 0 0 0;0 0 0 0 0 0;0 0 0 0 0 0;0 0 0 0 0 0;0 0 0 0 pitch_damping 0;0 0 0 0 0 0;]  Multiplication=Matrix(K*u) (u vector)
  "gravity 3dof {n}" : Subsystem
  invM_total : Constant  Value=invM_total
  "position of connection point to the Tugline1{b} [3 X n_tagline]" : Constant  Value=posTuggerline_b(:,1)
  "position of connection point to the Tuglines2{b} [3 X 1]" : Constant  Value=posTuggerline_b(:,2)
  "position of connection point to the lift sling1{b}" : Constant  Value=posSling_b(:,1)
  "position of connection point to the lift sling1{b}1" : Constant  Value=posSling_b(:,4)
  "position of connection point to the lift sling2{b}" : Constant  Value=posSling_b(:,2)
  "position of connection point to the lift sling2{b}1" : Constant  Value=posSling_b(:,3)
  "eta(6DOF){n}" : Outport
  "nu(6DOF){bb}" : Outport  Port=2
  BUS : Outport  Port=3
  wires:
  [eta_n] -> Bus Creator/16  "eta_n"
  Selector2/1 -> [p_n]
  "External force(3DOF){n} nu{b} to Force&Torque(6DOF){b}"/1 -> Sum3/4
  Sum/1 -> Sum1/1  "force and torque 6dof {bb}"
  Coriolis matrix at COG  [6X6]/1(Coriolis matrix 6X6) -> Divide1/1
  Divide1/1 -> Sum/4  "Coriolis force(6dof){b}"
  Divide/1 -> Integrator/1  "nu_dot{bb} = inv(M)*f_ex_bb"
  bladePar.totalMass+m_yoke/1 -> "gravity 3dof {n}"/1(mass), Coriolis matrix at COG  [6X6]/1(mass)
  bladePar.I_COG/1 -> Coriolis matrix at COG  [6X6]/2(I_COG)
  "Force(3DOF){b}2Force&Torque(6DOF){b}"/1 -> Sum/3  "gravity(6DOF){b}"
  "gravity 3dof {n}"/1("gravity{n}") -> "Translate velocity&force {n}2{b}"/2  "gravity {n}"
  6 DOF transformation for blade (z-x-y)/1 -> Integrator1/1, Selector1/1  "eta_dot(6DOF) {n}"
  "f_sling1{n} [3 X 1]"/1 -> "External force(3DOF){n} nu{b} to Force&Torque(6DOF){b}1"/2
  "Translate velocity&force {n}2{b}"/1 -> "Force(3DOF){b}2Force&Torque(6DOF){b}"/2  "gravity(3DOF){b}"
  bladePar.posCOG/1 -> "Force(3DOF){b}2Force&Torque(6DOF){b}"/1
  invM_total/1 -> Divide/1
  "position of connection point to the lift sling1{b}"/1 -> "External force(3DOF){n} nu{b} to Force&Torque(6DOF){b}1"/1
  "position of connection point to the Tugline1{b} [3 X n_tagline]"/1 -> "External force(3DOF){n} nu{b} to Force&Torque(6DOF){b}2"/1
  "f_tagline1{n} [3 X 1]"/1 -> "External force(3DOF){n} nu{b} to Force&Torque(6DOF){b}2"/2
  "External force(3DOF){n} nu{b} to Force&Torque(6DOF){b}2"/1 -> Sum2/2
  "tau_wind{bb}"/1 -> Sum1/2
  Sum1/1 -> Divide/2
  Selector1/1 -> [v_n]
  [p_n] -> Bus Creator/2  "p_n"
  [nu_b] -> Bus Creator/1  "nu_b"
  "External force(3DOF){n} nu{b} to Force&Torque(6DOF){b}1"/2 -> [posLiftwire1_n]
  [p_i_n] -> Bus Creator/4  "p_i_n"
  [posLiftwire1_n] -> Bus Creator/6  "posLiftwire1_n"
  [v_n] -> Bus Creator/3  "v_n"
  Bus Creator/1 -> BUS/1
  [posTugline1_n] -> Bus Creator/10  "posTugline1_n"
  "External force(3DOF){n} nu{b} to Force&Torque(6DOF){b}2"/2 -> [posTugline1_n]
  "External force(3DOF){n} nu{b} to Force&Torque(6DOF){b}1"/1 -> Sum3/3
  Sum2/1 -> Sum/1  "tau_tagline"
  "position of connection point to the Tuglines2{b} [3 X 1]"/1 -> "External force(3DOF){n} nu{b} to Force&Torque(6DOF){b}3"/1(pos_b)
  "f_tagline2{b} [3 X n_tagline]"/1 -> "External force(3DOF){n} nu{b} to Force&Torque(6DOF){b}3"/2("f_ex{b} [3 X n]")
  "External force(3DOF){n} nu{b} to Force&Torque(6DOF){b}3"/1(tau_ex [6n X 1]) -> Sum2/1
  "External force(3DOF){n} nu{b} to Force&Torque(6DOF){b}3"/2(pos_n[3 X 1]) -> [posTugline2_n]
  [posTugline2_n] -> Bus Creator/12  "posTugline2_n"
  "External force(3DOF){n} nu{b} to Force&Torque(6DOF){b}3"/3(nu_n[3 X 1]) -> [nuTugline2_n]
  "External force(3DOF){n} nu{b} to Force&Torque(6DOF){b}2"/3 -> [nuTugline1_n]
  "External force(3DOF){n} nu{b} to Force&Torque(6DOF){b}1"/3 -> [nuLiftwire1_n]
  [nuLiftwire1_n] -> Bus Creator/7  "nuLiftwire1_n"
  [nuTugline1_n] -> Bus Creator/11  "nuTugline1_n"
  [nuTugline2_n] -> Bus Creator/13  "nuTugline2_n"
  Sum3/1 -> Sum/2  "tau_sling"
  "f_sling2{n} [3 X 1]"/1 -> "External force(3DOF){n} nu{b} to Force&Torque(6DOF){b}"/2
  "position of connection point to the lift sling2{b}"/1 -> "External force(3DOF){n} nu{b} to Force&Torque(6DOF){b}"/1
  "External force(3DOF){n} nu{b} to Force&Torque(6DOF){b}"/2 -> [posLiftwire2_n]
  "External force(3DOF){n} nu{b} to Force&Torque(6DOF){b}"/3 -> [nuLiftwire2_n]
  "For Each pos{b} nu{b}  to pos{n}1"/1 -> [p_i_n]
  "For Each pos{b} nu{b}  to pos{n}1"/2 -> [nu_i_n]
  [nu_i_n] -> Bus Creator/5  "nu_i_n"
  [posLiftwire2_n] -> Bus Creator/8  "posLiftwire2_n"
  [nuLiftwire2_n] -> Bus Creator/9  "nuLiftwire2_n"
  "bladePar.posC_14_i{b}"/1 -> "For Each pos{b} nu{b}  to pos{n}1"/1
  "bladePar.posCenterLine_i{b}"/1 -> "For Each pos{b} nu{b}  to pos{n}"/1
  "For Each pos{b} nu{b}  to pos{n}"/2 -> [nuCenterLine_i_n]
  "For Each pos{b} nu{b}  to pos{n}"/1 -> [pCenterLine_i_n]
  [pCenterLine_i_n] -> Bus Creator/14  "pCenterLine_i_n"
  [nuCenterLine_i_n] -> Bus Creator/15  "nuCenterLine_i_n"
  Integrator/1 -> damping/1, "For Each pos{b} nu{b}  to pos{n}"/3, "For Each pos{b} nu{b}  to pos{n}1"/3, "nu(6DOF){bb}"/1, [nu_b], "External force(3DOF){n} nu{b} to Force&Torque(6DOF){b}4"/4, "External force(3DOF){n} nu{b} to Force&Torque(6DOF){b}5"/4, "External force(3DOF){n} nu{b} to Force&Torque(6DOF){b}2"/4, "External force(3DOF){n} nu{b} to Force&Torque(6DOF){b}3"/4("nu{b}"), "External force(3DOF){n} nu{b} to Force&Torque(6DOF){b}1"/4, "External force(3DOF){n} nu{b} to Force&Torque(6DOF){b}"/4, Coriolis matrix at COG  [6X6]/3("nu(6DOF){b}"), Divide1/2, 6 DOF transformation for blade (z-x-y)/2  "nu(6DOF){bb}"
  Integrator1/1 -> "For Each pos{b} nu{b}  to pos{n}"/2, "For Each pos{b} nu{b}  to pos{n}1"/2, "External force(3DOF){n} nu{b} to Force&Torque(6DOF){b}5"/3, "External force(3DOF){n} nu{b} to Force&Torque(6DOF){b}2"/3, "External force(3DOF){n} nu{b} to Force&Torque(6DOF){b}3"/3("eta{n}"), "External force(3DOF){n} nu{b} to Force&Torque(6DOF){b}4"/3, "External force(3DOF){n} nu{b} to Force&Torque(6DOF){b}1"/3, "External force(3DOF){n} nu{b} to Force&Torque(6DOF){b}"/3, "Translate velocity&force {n}2{b}"/1, 6 DOF transformation for blade (z-x-y)/1, Selector2/1, [eta_n], "eta(6DOF){n}"/1  "eta(6DOF){n}"
  "External force(3DOF){n} nu{b} to Force&Torque(6DOF){b}4"/3 -> [nuLiftwire3_n]
  "External force(3DOF){n} nu{b} to Force&Torque(6DOF){b}4"/2 -> [posLiftwire3_n]
  "position of connection point to the lift sling2{b}1"/1 -> "External force(3DOF){n} nu{b} to Force&Torque(6DOF){b}4"/1
  "f_sling3{n} [3 X 1]"/1 -> "External force(3DOF){n} nu{b} to Force&Torque(6DOF){b}4"/2
  "External force(3DOF){n} nu{b} to Force&Torque(6DOF){b}5"/3 -> [nuLiftwire4_n]
  "External force(3DOF){n} nu{b} to Force&Torque(6DOF){b}5"/1 -> Sum3/1
  "External force(3DOF){n} nu{b} to Force&Torque(6DOF){b}5"/2 -> [posLiftwire4_n]
  "position of connection point to the lift sling1{b}1"/1 -> "External force(3DOF){n} nu{b} to Force&Torque(6DOF){b}5"/1
  "f_sling4{n} [3 X 1]"/1 -> "External force(3DOF){n} nu{b} to Force&Torque(6DOF){b}5"/2
  "External force(3DOF){n} nu{b} to Force&Torque(6DOF){b}4"/1 -> Sum3/2
  [nuLiftwire4_n] -> Bus Creator/20  "nuLiftwire4_n"
  [posLiftwire4_n] -> Bus Creator/19  "posLiftwire4_n"
  [nuLiftwire3_n] -> Bus Creator/18  "nuLiftwire3_n"
  [posLiftwire3_n] -> Bus Creator/17  "posLiftwire3_n"
  damping/1 -> Sum1/3

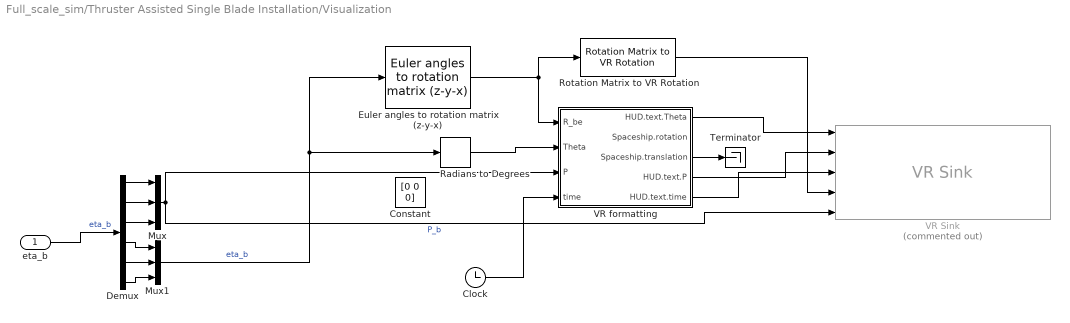
== system Full_scale_sim/Thruster Assisted Single Blade Installation/Visualization ==
  eta_b : Inport
  Clock : Clock
  Constant : Constant  Value=[0 0 0]
  Demux : Demux  Outputs=6
  Euler angles to rotation matrix (z-y-x) : MarIn_blade/Basic functions/Euler angles to rotation matrix (z-y-x)
      settings: SourceProductName=MarIn (Blade)
  Mux : Mux  Inputs=3
  Mux1 : Mux  Inputs=3
  Radians to Degrees : simulink_extras/Transformations/Radians to Degrees
  Rotation Matrix to VR Rotation : vrlib/Utilities/Rotation Matrix to VR Rotation  maxzero=1e-12
  Terminator : Terminator
  VR Sink : vrlib/VR Sink  Commented=on  InstantiateOnLoad=on  SampleTime=.1  ViewEnable=on  RemoteChange=off  RemoteView=off  FieldsWritten=HUDText1.string.1.-1.1.char#HUDTextPos.string.1.-1.1.char#HUDTextTime.string.1.-1.1.char#Blade_IEA-15-240-RWT.rotation.4.1.1.double#Blade_IEA-15-240-RWT.translation.3.1.1.double  WorldFileName=C:\Users\sstor\Syddansk Universitet\Bachelor Tobias&Seb - General\Simulink\Visualization_blade_v2\spaceship_VR.x3d  WorldDescription=VR Spaceship Dragon  AutoView=off  VideoDimensions=[]  AllowVariableSize=off  FigureProperties=[]
  VR formatting : Subsystem
  wires:
  Euler angles to rotation matrix (z-y-x)/1 -> VR formatting/1(R_be), Rotation Matrix to VR Rotation/1
  Mux1/1 -> Euler angles to rotation matrix (z-y-x)/1, Radians to Degrees/1  "eta_b"
  VR formatting/3(Spaceship.translation) -> Terminator/1
  eta_b/1 -> Demux/1  "eta_b"
  Demux/4 -> Mux1/1
  Demux/5 -> Mux1/2
  Demux/6 -> Mux1/3
  Demux/1 -> Mux/1
  Demux/2 -> Mux/2
  Demux/3 -> Mux/3
  Radians to Degrees/1 -> VR formatting/2(Theta)
  Mux/1 -> VR Sink/5, VR formatting/3(P)  "P_b"
  VR formatting/1(HUD.text.Theta) -> VR Sink/1
  VR formatting/4(HUD.text.P) -> VR Sink/2
  Rotation Matrix to VR Rotation/1 -> VR Sink/4
  Clock/1 -> VR formatting/4(time)
  VR formatting/5(HUD.text.time) -> VR Sink/3

== system Full_scale_sim/Thruster Assisted Single Blade Installation/wind ramp2 ==
  Demux : Demux  Tag=STV Demux  Outputs=1
      settings: DisplayOption=none
  FromWs : FromWorkspace  Tag=STV FromWs  VariableName=tuvar
      SigBuilderData=|
      | common.afterFinalStr = 'Extrapolate'
      | common.sampleTime = 0
      | dataSet.timeRange = [0 3000]
      | dataSet.name = 'Group 1'
      | sbobj.Groups.Name = 'Group 1'
      | sbobj.Groups.Signals.Name = 'Signal 1'
      | sbobj.Groups.Signals.XData = [0 1 3000]
      | sbobj.Groups.Signals.YData = [0 1 1]
      | sbobj.Groups.TimeRange = [0 3000]
  Signal 1 : Outport  Tag=STV Outport
  wires:
  Demux/1 -> Signal 1/1
  FromWs/1 -> Demux/1

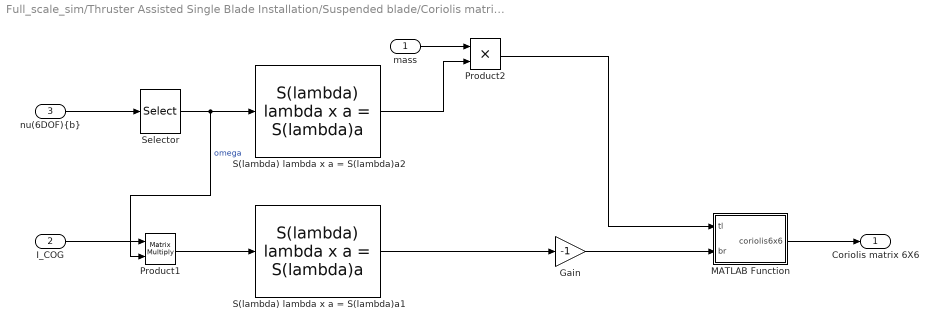
== system Full_scale_sim/Thruster Assisted Single Blade Installation/Suspended blade/Coriolis matrix at COG  [6X6] ==
  mass : Inport
  I_COG : Inport  Port=2
  "nu(6DOF){b}" : Inport  Port=3
  Gain : Gain  Gain=-1
  MATLAB Function : MATLAB Function  TreatAsAtomicUnit=on
  Product1 : Product  Multiplication=Matrix(*)
  Product2 : Product
  S(lambda) lambda x a = S(lambda)a1 : MarIn_blade/Basic functions/S(lambda) lambda x a = S(lambda)a
      settings: SourceProductName=MarIn(Blade)
  S(lambda) lambda x a = S(lambda)a2 : MarIn_blade/Basic functions/S(lambda) lambda x a = S(lambda)a
      settings: SourceProductName=MarIn(Blade)
  Selector : Selector  InputPortWidth=6  IndexOptions=Index vector (dialog)  Indices=[1 2 3]  OutputSizes=1
  Coriolis matrix 6X6 : Outport
  wires:
  Selector/1 -> Product1/2, S(lambda) lambda x a = S(lambda)a2/1  "omega"
  Gain/1 -> MATLAB Function/2(br)
  MATLAB Function/1(coriolis6x6) -> Coriolis matrix 6X6/1
  S(lambda) lambda x a = S(lambda)a1/1 -> Gain/1
  Product2/1 -> MATLAB Function/1(tl)
  "nu(6DOF){b}"/1 -> Selector/1
  I_COG/1 -> Product1/1
  mass/1 -> Product2/1
  S(lambda) lambda x a = S(lambda)a2/1 -> Product2/2
  Product1/1 -> S(lambda) lambda x a = S(lambda)a1/1
